simulink model "SimscapeCrane_MPCsoft"  (R2016a)
settings: Solver=ode15s  StartTime=0.0  StopTime=""  RelTol=1e-3
values from neighbouring files (symbols this model uses):
  bb = randn(2 * N * (c + m), 1)    [compare.m]    (also in test.m; testMyMPC.m = bs)
  F = randn(2 * N * (c + m), N * m)    [compare.m]    (also in test.m; testMyMPC.m = Fs)
  gs = rho * ones(N*c, 1)    [mySoftPadding.m]
  H = randn(N * m , N * m)    [compare.m]    (also in test.m; testMyMPC.m = H\eye(size(H)))
  J = randn(2 * N * (c + m), n)    [compare.m]    (also in test.m; testMyMPC.m = Js)
  L = randn(2 * N * (c + m), n)    [compare.m]    (also in test.m; testMyMPC.m = Ls)
  m = 2    [compare.m]    (also in test.m)
  N = 5    [compare.m]    (also in mySoftPadding.m = size(H, 2)/m; test.m; testMyMPC.m = ceil(Tf/Ts))
  Ts = 1/10    (= 0.1)    [testMyMPC.m]
  xTarget = 0.8*[xRange(2) 0 yRange(2) 0 0 0 0 0]'    [testMyMPC.m]
  xZero = xRange(1)    [testMyMPC.m]
  yZero = yRange(1)    [testMyMPC.m]
undefined symbols (not defined in the file or in its folder): G, MR, TxBreak, TxCoulomb, TxVisc, TyBreak, TyCoulomb, TzBreak, TzCoulomb, X, xRange, Y, yRange, Z, zRange, zZero
undefined symbols (not defined in the file): M, TorqueMultX, TorqueMultY, TorqueMultZ, TxTrans, TyTrans, TyVisc, TzTrans, TzVisc
libraries: sm_lib x146, fl_lib x62, nesl_utility x24, elec_lib x9, simulink x6, sm_double_wishbone_suspension_lib x4, aerolibtransform2 x1
(part 1 of 14)
settings Model: Creator=jsustare  LastModifiedBy=acrisne
settings SolverCC: MaxConsecutiveMinStep=10
settings DataIOCC: SaveFormat=StructureWithTime
settings DebuggingCC: AllowSymbolicDim=off
settings ModelReferenceCC: PropagateSignalLabelsOutOfModel=off
settings GRTTargetCC: GeneratePreprocessorConditionals=Use local settings
settings ConfigurationSet: Description=SimMechanics 2G

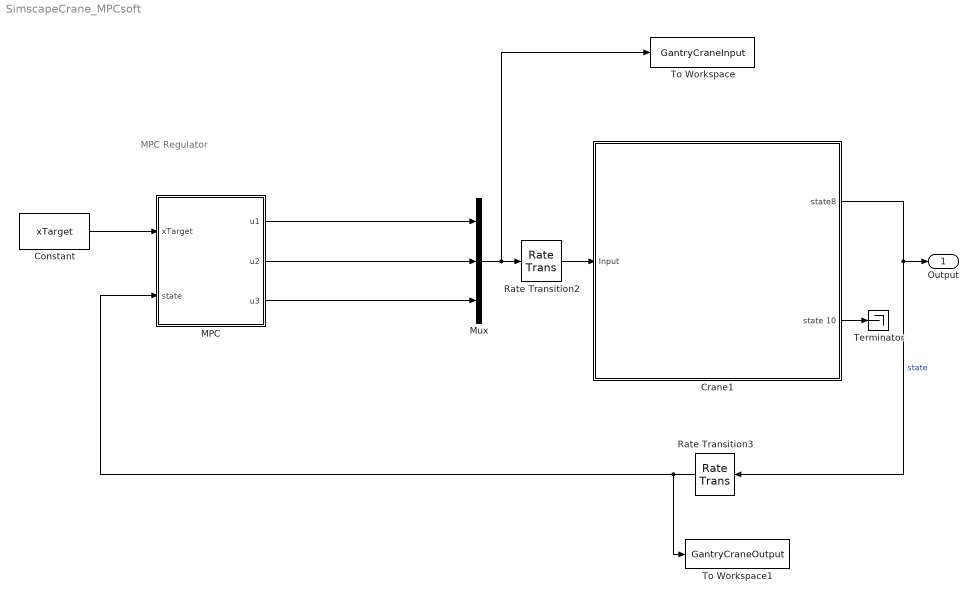
== system SimscapeCrane_MPCsoft ==
  note: MPC Regulator
  Constant : Constant  Value=xTarget
  Crane1 : Subsystem  mask{penduMass=m, cartMass=M, MR=MR, xRange=xRange, yRange=yRange, zRange=zRange, xZero=xZero, yZero=yZero, zZero=zZero, TxBreak=TxBreak, TxCoulomb=TxCoulomb, TxVisc=TxVisc, TxTrans=TxTrans, TyBreak=TyBreak, TyCoulomb=TyCoulomb, TyVisc=TyVisc, TyTrans=TyTrans, TzBreak=TzBreak, TzCoulomb=TzCoulomb, TzVisc=TzVisc, TzTrans=TzTrans, Ux=TorqueMultX, Uy=TorqueMultY, Uz=TorqueMultZ}
      mask prompts: penduMass "Pendulum Mass (Kg)"; cartMass "Mass of the cart (Kg)"; MR "Mass of the rail (Kg)"; TxBreak "BreakAwayFriction"; TxCoulomb "Coulomb Friction"; TxVisc "Viscous friction"; TxTrans "Transition coeff"; TyBreak "BreakAwayFriction"; TyCoulomb "Coulomb Friction"; TyVisc "Viscous friction"; TyTrans "Transition coeff"; TzBreak "BreakAwayFriction"; TzCoulomb "Coulomb Friction"; TzVisc "Viscous friction"; TzTrans "Transition coeff"; Ux "Rail motor multiplier (X)"; Uy "Cart motor multiplier (Y)"; Uz "String motor multiplier (Z)"
      mask init:
      | %mass lowSat
      | penduMass=max(penduMass,1e-3);
      | cartMass=max(cartMass,1e-3);
      | MR=max(MR,1e-3);
      | 
      | %zeros saturated
      | xZero=max(xZero,xRange(1));
      | xZero=min(xZero,xRange(2));
      | 
      | yZero=max(yZero,yRange(1));
      | yZero=min(yZero,yRange(2));
      | 
      | zZero=max(zZero,zRange(1));
      | zZero=min(zZero,zRange(2));
      mask DialogControl DescGroupVar Prompt: 3D Crane Simscape model
      mask Display:
